simulink model "sh_plant"  (R2021b)
settings: Solver=VariableStepAuto  StartTime=0.0  StopTime=10.0  RelTol=1e-3
model workspace (MAT data in the model file):
  i = 2
values from neighbouring files (symbols this model uses):
  c_h = 6e03    (= 6000)    [skyhook.m]
  c_l = 1.5e03    (= 1500)    [skyhook.m]
  k1 = 29e03    (= 29000)    [skyhook.m]
  k2 = 228e03    (= 228000)    [skyhook.m]
  m1 = 380    [skyhook.m]
  m2 = 31    [skyhook.m]
  passive_damping = c_h    (= 6000)    [skyhook.m]
  semi_active = 0    [skyhook.m]
settings Model: Creator=DAUIN-Win10  LastModifiedBy=Luca

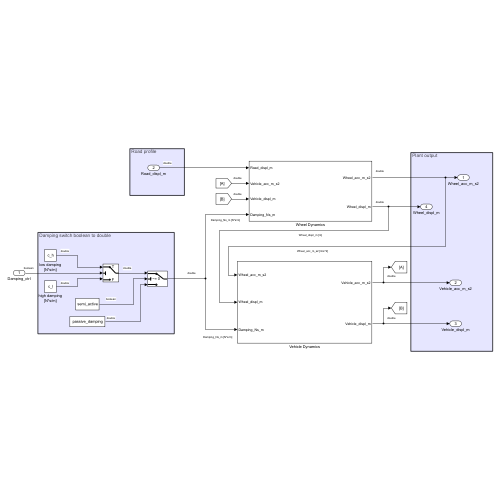
[thumbnail: Simulink's stored preview of the top-level diagram]
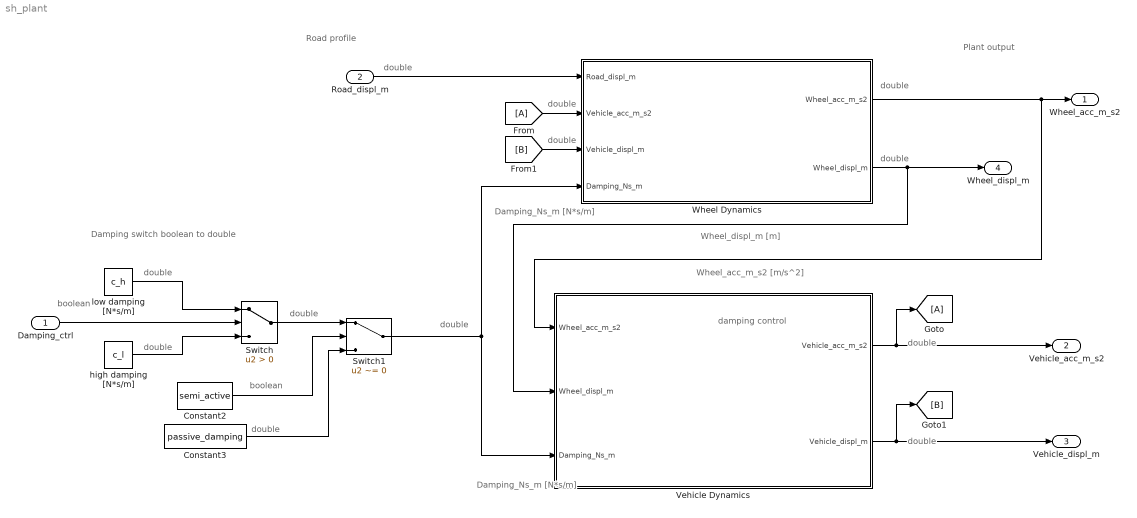
== system sh_plant ==
  note: double
  note: Damping switch boolean to double
  note: damping control
  note: Road profile
  note: Plant output
  note: boolean
  note: boolean
  note: double
  note: Wheel_displ_m [m]
  note: Wheel_acc_m_s2 [m/s^2]
  note: Damping_Ns_m [N*s/m]
  note: Damping_Ns_m [N*s/m]
  note: double
  note: double
  note: double
  note: double
  note: double
  note: double
  note: double
  note: double
  note: double
  note: double
  Damping_ctrl : Inport  OutDataTypeStr=boolean
  Road_displ_m : Inport  Port=2  OutDataTypeStr=double
  Constant2 : Constant  Description=boolean  Value=semi_active  OutDataTypeStr=boolean
  Constant3 : Constant  Value=passive_damping
  Switch : Switch  Criteria=u2 > Threshold
  Switch1 : Switch  Criteria=u2 ~= 0
  Vehicle Dynamics : Subsystem
  Wheel Dynamics : Subsystem
  high damping [N*s/m] : Constant  Value=c_l
  low damping [N*s/m] : Constant  Value=c_h
  Wheel_acc_m_s2 : Outport
  Vehicle_acc_m_s2 : Outport  Port=2
  Vehicle_displ_m : Outport  Port=3
  Wheel_displ_m : Outport  Port=4
  wires:
  Road_displ_m/1 -> Wheel Dynamics/1(Road_displ_m)
  Wheel Dynamics/1(Wheel_acc_m_s2) -> Vehicle Dynamics/1(Wheel_acc_m_s2), Wheel_acc_m_s2/1
  Wheel Dynamics/2(Wheel_displ_m) -> Wheel_displ_m/1, Vehicle Dynamics/2(Wheel_displ_m)
  Vehicle Dynamics/2(Vehicle_displ_m) -> Vehicle_displ_m/1, [B]
  Vehicle Dynamics/1(Vehicle_acc_m_s2) -> [A], Vehicle_acc_m_s2/1
  [A] -> Wheel Dynamics/2(Vehicle_acc_m_s2)
  [B] -> Wheel Dynamics/3(Vehicle_displ_m)
  high damping [N*s/m]/1 -> Switch/3
  Damping_ctrl/1 -> Switch/2
  low damping [N*s/m]/1 -> Switch/1
  Switch/1 -> Switch1/1
  Constant2/1 -> Switch1/2
  Constant3/1 -> Switch1/3
  Switch1/1 -> Wheel Dynamics/4(Damping_Ns_m), Vehicle Dynamics/3(Damping_Ns_m)

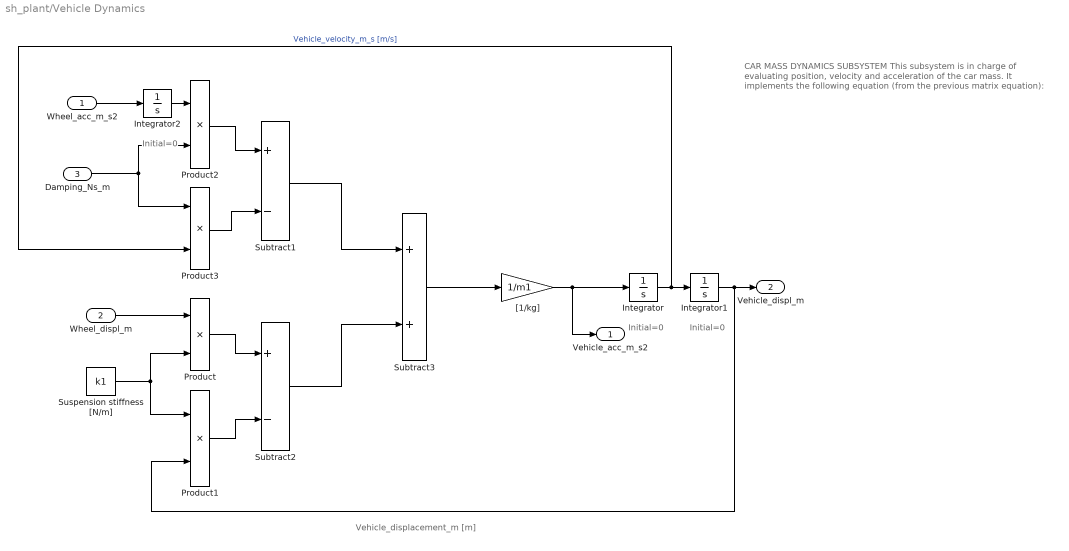
== system sh_plant/Vehicle Dynamics ==
  note: Vehicle_displacement_m [m]
  note: CAR MASS DYNAMICS SUBSYSTEM
      | This subsystem is in charge of evaluating position,
      | velocity and acceleration of the car mass.
      | It implements the following equation (from the previous
      | matrix equation):
  note: Initial=0
  note: Initial=0
  note: Initial=0
  Wheel_acc_m_s2 : Inport
  Wheel_displ_m : Inport  Port=2
  Damping_Ns_m : Inport  Port=3
  Integrator : Integrator
  Integrator1 : Integrator
  Integrator2 : Integrator
  Product{,1..3} (4 alike) : Product
  Subtract1 : Sum  Inputs=+-
  Subtract2 : Sum  Inputs=+-
  Subtract3 : Sum
  Suspension stiffness [N/m] : Constant  Value=k1
  "[1/kg]" : Gain  Gain=1/m1
  Vehicle_acc_m_s2 : Outport
  Vehicle_displ_m : Outport  Port=2
  wires:
  Suspension stiffness [N/m]/1 -> Product1/1, Product/2
  "[1/kg]"/1 -> Vehicle_acc_m_s2/1, Integrator/1
  Wheel_displ_m/1 -> Product/1
  Integrator/1 -> Product3/2, Integrator1/1  "Vehicle_velocity_m_s [m/s]"
  Integrator1/1 -> Product1/2, Vehicle_displ_m/1
  Wheel_acc_m_s2/1 -> Integrator2/1
  Integrator2/1 -> Product2/1
  Damping_Ns_m/1 -> Product3/1, Product2/2
  Product2/1 -> Subtract1/1
  Product3/1 -> Subtract1/2
  Product/1 -> Subtract2/1
  Product1/1 -> Subtract2/2
  Subtract3/1 -> "[1/kg]"/1
  Subtract1/1 -> Subtract3/1
  Subtract2/1 -> Subtract3/2

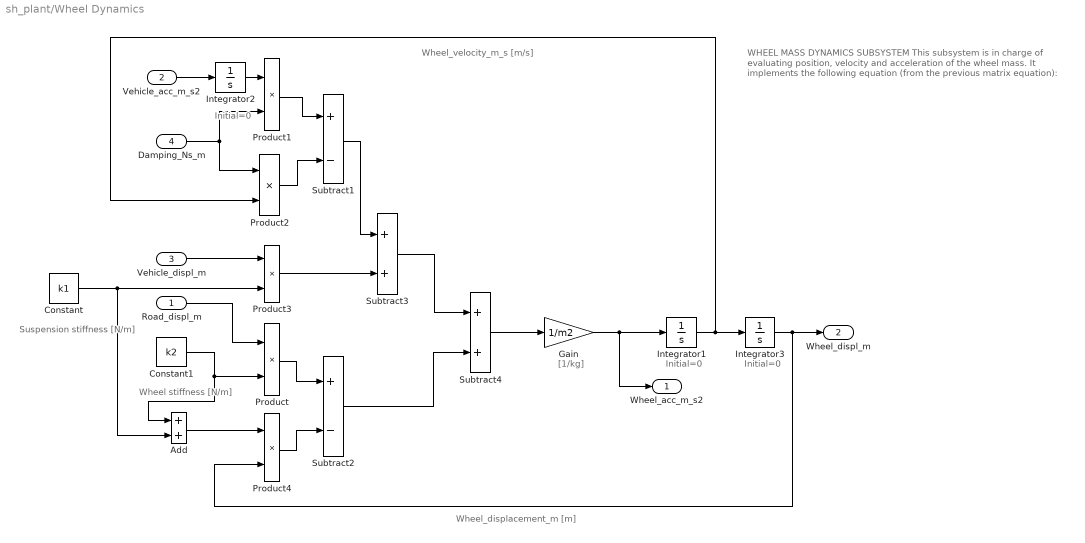
== system sh_plant/Wheel Dynamics ==
  note: Wheel_displacement_m [m]
  note: Initial=0
  note: WHEEL MASS DYNAMICS SUBSYSTEM
      | This subsystem is in charge of evaluating position, velocity
      | and acceleration of the wheel mass.
      | It implements the following equation (from the previous
      | matrix equation):
  note: Initial=0
  note: Initial=0
  note: [1/kg]
  note: Wheel stiffness
      | [N/m]
  note: Suspension stiffness
      | [N/m]
  note: Wheel_velocity_m_s [m/s]
  Road_displ_m : Inport
  Vehicle_acc_m_s2 : Inport  Port=2
  Vehicle_displ_m : Inport  Port=3
  Damping_Ns_m : Inport  Port=4
  Add : Sum
  Constant : Constant  Value=k1
  Constant1 : Constant  Value=k2
  Gain : Gain  Gain=1/m2
  Integrator1 : Integrator
  Integrator2 : Integrator
  Integrator3 : Integrator
  Product{,1..4} (5 alike) : Product
  Subtract1 : Sum  Inputs=+-
  Subtract2 : Sum  Inputs=+-
  Subtract3 : Sum
  Subtract4 : Sum
  Wheel_acc_m_s2 : Outport
  Wheel_displ_m : Outport  Port=2
  wires:
  Gain/1 -> Integrator1/1, Wheel_acc_m_s2/1
  Integrator3/1 -> Wheel_displ_m/1, Product4/2
  Integrator1/1 -> Integrator3/1, Product2/2
  Vehicle_displ_m/1 -> Product3/1
  Vehicle_acc_m_s2/1 -> Integrator2/1
  Constant/1 -> Product3/2, Add/2
  Add/1 -> Product4/1
  Road_displ_m/1 -> Product/1
  Constant1/1 -> Add/1, Product/2
  Damping_Ns_m/1 -> Product2/1, Product1/2
  Product1/1 -> Subtract1/1
  Product2/1 -> Subtract1/2
  Product4/1 -> Subtract2/2
  Product/1 -> Subtract2/1
  Product3/1 -> Subtract3/2
  Subtract1/1 -> Subtract3/1
  Subtract4/1 -> Gain/1
  Subtract2/1 -> Subtract4/2
  Subtract3/1 -> Subtract4/1
  Integrator2/1 -> Product1/1
